simulink model "Lab2Task2"  (R2020a)
settings: Solver=VariableStepAuto  StartTime=0.0  StopTime=2  RelTol=1e-3
libraries: powerlib x15
settings Model: Creator=Dell  LastModifiedBy=Dell

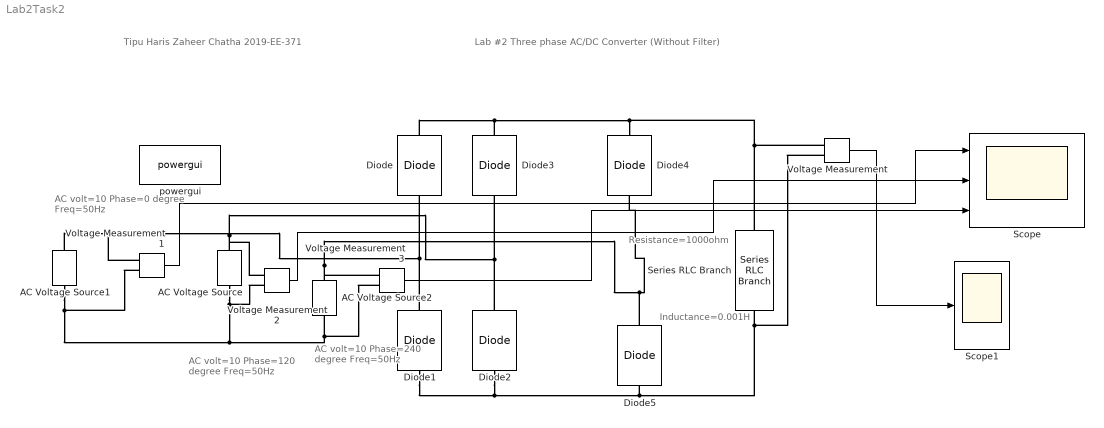
== system Lab2Task2 ==
  note: Inductance=0.001H
  note: AC volt=10
      | Phase=240 degree
      | Freq=50Hz
  note: Resistance=1000ohm
  note: AC volt=10
      | Phase=120 degree
      | Freq=50Hz
  note: Lab #2
      | Three phase AC/DC Converter (Without Filter)
  note: Tipu Haris Zaheer Chatha
      | 2019-EE-371
  note: AC volt=10
      | Phase=0 degree
      | Freq=50Hz
  AC Voltage Source : powerlib/Electrical Sources/AC Voltage Source  Amplitude=10  Phase=120  Frequency=50  SampleTime=0  Measurements=None  BusType=swing  Pref=10e3  Qref=0  Qmin=-inf  Qmax=+inf
  AC Voltage Source1 : powerlib/Electrical Sources/AC Voltage Source  Amplitude=10  Phase=0  Frequency=50  SampleTime=0  Measurements=None  BusType=swing  Pref=10e3  Qref=0  Qmin=-inf  Qmax=+inf
  AC Voltage Source2 : powerlib/Electrical Sources/AC Voltage Source  Amplitude=10  Phase=240  Frequency=50  SampleTime=0  Measurements=None  BusType=swing  Pref=10e3  Qref=0  Qmin=-inf  Qmax=+inf
  Diode{,1..5} (6 alike) : powerlib/Power Electronics/Diode  Ron=0.001  Lon=0  Vf=0.8  IC=0  UseSnubber=0  Rs=500  Cs=250e-9  Measurements=off
  Scope : Scope  NumInputPorts=3
  Scope1 : Scope
  Series RLC Branch : powerlib/Elements/Series RLC Branch  LConnTagsString=__new0  RConnTagsString=__new0  BranchType=R  Resistance=1000  Inductance=1e-3  SetiL0=off  InitialCurrent=0  Capacitance=1e-6  Setx0=off  InitialVoltage=0  Measurements=None
  Voltage Measurement{,1..3} (4 alike) : powerlib/Measurements/Voltage Measurement  PhasorSimulation=off  OutputType=Complex  PSBequivalent=0
  powergui : powerlib/powergui  Priority=1  SimulationMode=Discrete  SampleTime=50e-6  frequency=60  Iterations=50  frequencyindice=50  Pbase=100e6  ErrMax=1e-4  UnitsV=kV  UnitsW=MW  buscounter=0  FunctionMessages=off  echomessages=off  EnableUseOfTLC=off  CurrentSourceSwitches=off  DisableSnubberDevices=off  DisableRonSwitches=off  DisableVfSwitches=off  DisplayEquations=off  AutomaticDiscreteSolvers=off  SolverType=Tustin/Backward Euler (TBE)  Interpol=off  ExternalGateDelay=off  methode=off  Ts=100  x0status=blocks  SPID=on  SwTol=0  HookPort=off  NonlinearTolerance=1e-4  nMaxIteration=100  ContinueOnMaxIteration=off  RestoreLinks=warning  ResistiveCurrentMeasurement=off  Frange=[0:2:500]  Ylog=off  Xlog=on  ShowGrid=off  save=off  variable=ZData  structure=0  ZoomFFT=off  StartTime=0.0  cycles=1  DisplayStyle=1  fundamental=60  FreqAxis=off  MaxFrequency=1000  frequencyindicesteady=1  RmsSteady=1  display=off
  wires:
  Voltage Measurement1/1 -> Scope/1
  Voltage Measurement2/1 -> Scope/2
  Voltage Measurement3/1 -> Scope/3
  Voltage Measurement/1 -> Scope1/1
  connections:
  Diode2/RConn1 -- Diode3/LConn1 -- AC Voltage Source/RConn1 -- Voltage Measurement2/LConn1
  Diode2/LConn1 -- Diode1/LConn1 -- Voltage Measurement/LConn2 -- Series RLC Branch/RConn1 -- Diode5/LConn1
  AC Voltage Source2/RConn1 -- Diode4/LConn1 -- Diode5/RConn1 -- Voltage Measurement3/LConn1
  AC Voltage Source/LConn1 -- AC Voltage Source1/LConn1 -- Voltage Measurement1/LConn2 -- Voltage Measurement3/LConn2 -- AC Voltage Source2/LConn1 -- Voltage Measurement2/LConn2
  Diode4/RConn1 -- Series RLC Branch/LConn1 -- Voltage Measurement/LConn1 -- Diode3/RConn1 -- Diode/RConn1
  Voltage Measurement1/LConn1 -- Diode1/RConn1 -- Diode/LConn1 -- AC Voltage Source1/RConn1
